simulink model "test_FOPID"  (R2024a)
settings: Solver=VariableStepAuto  StartTime=0.0  StopTime=0.1  RelTol=1e-3
undefined symbols (not defined in the file or in its folder): control_a, control_p, force_a, force_p, rpm_a, rpm_p
libraries: fod x145, slpidlib x15
(part 4 of 4)

== system test_FOPID/FOPID/ISE/Subsystem/TRAS 2_dof model 2/r(x2,x6) ==
  y2 : Inport
  x6 : Inport  Port=2
  +2 : Sum  InputSameDT=on  SaturateOnIntegerOverflow=on  OutDataTypeStr=Inherit: Same as first input
  Mux : Mux  Inputs=2
  r2 : Fcn  Expr=- ( 0.0292*cos(u)+ 0.0546*sin(u))*1.7143
  s : Fcn  Expr="(u(1)^2)*(     -0.07389953104162*  0.28753198180218*sin(u(2))*cos(u(2)))"
  r : Outport
  wires:
  Mux/1 -> s/1
  r2/1 -> +2/1
  s/1 -> +2/2
  x6/1 -> Mux/2, r2/1
  +2/1 -> r/1
  y2/1 -> Mux/1

== system test_FOPID/FOPID/ITAE/Subsystem/TRAS 2_dof model 2/DCP-azimuth ==
  CTR_A : Inport
  1/Ja : Gain  Gain=37000  SaturateOnIntegerOverflow=on  OutDataTypeStr=Inherit: Same as input  ParamDataTypeStr=Inherit: Same as input
  CtrlA(rpma) : Lookup  InputValues=rpm_a  Table=control_a
  Integrator1 : Integrator
  Sum1 : Sum  Inputs=|+-  InputSameDT=on  SaturateOnIntegerOverflow=on  OutDataTypeStr=Inherit: Same as first input
  forceA(rpma) : Lookup  InputValues=rpm_a  Table=force_a
  RPM_A : Outport
  FORCE_A : Outport  Port=2
  wires:
  Sum1/1 -> Integrator1/1
  CtrlA(rpma)/1 -> Sum1/2
  Integrator1/1 -> 1/Ja/1
  1/Ja/1 -> CtrlA(rpma)/1, forceA(rpma)/1, RPM_A/1
  CTR_A/1 -> Sum1/1
  forceA(rpma)/1 -> FORCE_A/1

== system test_FOPID/FOPID/ITAE/Subsystem/TRAS 2_dof model 2/DCP_pith ==
  CTR_P : Inport
  1/Jp1 : Gain  Gain=6100  OutDataTypeStr=Inherit: Same as input  ParamDataTypeStr=Inherit: Same as input
  CtrlP(rpmp) : Lookup  InputValues=rpm_p  Table=control_p
  Integrator : Integrator
  Sum : Sum  Inputs=|+-  InputSameDT=on  SaturateOnIntegerOverflow=on  OutDataTypeStr=Inherit: Same as first input
  force(rpmp) : Lookup  InputValues=rpm_p  Table=force_p
  RPM_P : Outport
  FORCE_P : Outport  Port=2
  wires:
  Sum/1 -> Integrator/1
  Integrator/1 -> 1/Jp1/1
  CtrlP(rpmp)/1 -> Sum/2
  1/Jp1/1 -> RPM_P/1, CtrlP(rpmp)/1, force(rpmp)/1
  CTR_P/1 -> Sum/1
  force(rpmp)/1 -> FORCE_P/1

== system test_FOPID/FOPID/ITAE/Subsystem/TRAS 2_dof model 2/q (x2,x6) ==
  x2 : Inport
  x6 : Inport  Port=2
  " q(x6)" : Fcn  Expr=( (0.0268-0.00300962066650)*cos(u)^2) +0.00300962066650
  *1 : Product  Inputs=*/  InputSameDT=on  SaturateOnIntegerOverflow=on  OutDataTypeStr=Inherit: Same as first input
  q : Outport
  wires:
  *1/1 -> q/1
  x2/1 -> *1/1
  x6/1 -> " q(x6)"/1
  " q(x6)"/1 -> *1/2

== system test_FOPID/FOPID/ITAE/Subsystem/TRAS 2_dof model 2/r(x2,x6) ==
  y2 : Inport
  x6 : Inport  Port=2
  +2 : Sum  InputSameDT=on  SaturateOnIntegerOverflow=on  OutDataTypeStr=Inherit: Same as first input
  Mux : Mux  Inputs=2
  r2 : Fcn  Expr=- ( 0.0292*cos(u)+ 0.0546*sin(u))*1.7143
  s : Fcn  Expr="(u(1)^2)*(     -0.07389953104162*  0.28753198180218*sin(u(2))*cos(u(2)))"
  r : Outport
  wires:
  Mux/1 -> s/1
  r2/1 -> +2/1
  s/1 -> +2/2
  x6/1 -> Mux/2, r2/1
  +2/1 -> r/1
  y2/1 -> Mux/1

== system test_FOPID/FOPID/ITSE/Subsystem/TRAS 2_dof model 2/DCP-azimuth ==
  CTR_A : Inport
  1/Ja : Gain  Gain=37000  SaturateOnIntegerOverflow=on  OutDataTypeStr=Inherit: Same as input  ParamDataTypeStr=Inherit: Same as input
  CtrlA(rpma) : Lookup  InputValues=rpm_a  Table=control_a
  Integrator1 : Integrator
  Sum1 : Sum  Inputs=|+-  InputSameDT=on  SaturateOnIntegerOverflow=on  OutDataTypeStr=Inherit: Same as first input
  forceA(rpma) : Lookup  InputValues=rpm_a  Table=force_a
  RPM_A : Outport
  FORCE_A : Outport  Port=2
  wires:
  Sum1/1 -> Integrator1/1
  CtrlA(rpma)/1 -> Sum1/2
  Integrator1/1 -> 1/Ja/1
  1/Ja/1 -> CtrlA(rpma)/1, forceA(rpma)/1, RPM_A/1
  CTR_A/1 -> Sum1/1
  forceA(rpma)/1 -> FORCE_A/1

== system test_FOPID/FOPID/ITSE/Subsystem/TRAS 2_dof model 2/DCP_pith ==
  CTR_P : Inport
  1/Jp1 : Gain  Gain=6100  OutDataTypeStr=Inherit: Same as input  ParamDataTypeStr=Inherit: Same as input
  CtrlP(rpmp) : Lookup  InputValues=rpm_p  Table=control_p
  Integrator : Integrator
  Sum : Sum  Inputs=|+-  InputSameDT=on  SaturateOnIntegerOverflow=on  OutDataTypeStr=Inherit: Same as first input
  force(rpmp) : Lookup  InputValues=rpm_p  Table=force_p
  RPM_P : Outport
  FORCE_P : Outport  Port=2
  wires:
  Sum/1 -> Integrator/1
  Integrator/1 -> 1/Jp1/1
  CtrlP(rpmp)/1 -> Sum/2
  1/Jp1/1 -> RPM_P/1, CtrlP(rpmp)/1, force(rpmp)/1
  CTR_P/1 -> Sum/1
  force(rpmp)/1 -> FORCE_P/1

== system test_FOPID/FOPID/ITSE/Subsystem/TRAS 2_dof model 2/q (x2,x6) ==
  x2 : Inport
  x6 : Inport  Port=2
  " q(x6)" : Fcn  Expr=( (0.0268-0.00300962066650)*cos(u)^2) +0.00300962066650
  *1 : Product  Inputs=*/  InputSameDT=on  SaturateOnIntegerOverflow=on  OutDataTypeStr=Inherit: Same as first input
  q : Outport
  wires:
  *1/1 -> q/1
  x2/1 -> *1/1
  x6/1 -> " q(x6)"/1
  " q(x6)"/1 -> *1/2

== system test_FOPID/FOPID/ITSE/Subsystem/TRAS 2_dof model 2/r(x2,x6) ==
  y2 : Inport
  x6 : Inport  Port=2
  +2 : Sum  InputSameDT=on  SaturateOnIntegerOverflow=on  OutDataTypeStr=Inherit: Same as first input
  Mux : Mux  Inputs=2
  r2 : Fcn  Expr=- ( 0.0292*cos(u)+ 0.0546*sin(u))*1.7143
  s : Fcn  Expr="(u(1)^2)*(     -0.07389953104162*  0.28753198180218*sin(u(2))*cos(u(2)))"
  r : Outport
  wires:
  Mux/1 -> s/1
  r2/1 -> +2/1
  s/1 -> +2/2
  x6/1 -> Mux/2, r2/1
  +2/1 -> r/1
  y2/1 -> Mux/1

== system test_FOPID/FOPID/sensibility/Subsystem/TRAS 2_dof model 3/DCP-azimuth ==
  CTR_A : Inport
  1/Ja : Gain  Gain=37000  SaturateOnIntegerOverflow=on  OutDataTypeStr=Inherit: Same as input  ParamDataTypeStr=Inherit: Same as input
  CtrlA(rpma) : Lookup  InputValues=rpm_a  Table=control_a
  Integrator1 : Integrator
  Sum1 : Sum  Inputs=|+-  InputSameDT=on  SaturateOnIntegerOverflow=on  OutDataTypeStr=Inherit: Same as first input
  forceA(rpma) : Lookup  InputValues=rpm_a  Table=force_a
  RPM_A : Outport
  FORCE_A : Outport  Port=2
  wires:
  forceA(rpma)/1 -> FORCE_A/1
  CTR_A/1 -> Sum1/1
  1/Ja/1 -> RPM_A/1, forceA(rpma)/1, CtrlA(rpma)/1
  Integrator1/1 -> 1/Ja/1
  CtrlA(rpma)/1 -> Sum1/2
  Sum1/1 -> Integrator1/1

== system test_FOPID/FOPID/sensibility/Subsystem/TRAS 2_dof model 3/DCP_pith ==
  CTR_P : Inport
  1/Jp1 : Gain  Gain=6100  OutDataTypeStr=Inherit: Same as input  ParamDataTypeStr=Inherit: Same as input
  CtrlP(rpmp) : Lookup  InputValues=rpm_p  Table=control_p
  Integrator : Integrator
  Sum : Sum  Inputs=|+-  InputSameDT=on  SaturateOnIntegerOverflow=on  OutDataTypeStr=Inherit: Same as first input
  force(rpmp) : Lookup  InputValues=rpm_p  Table=force_p
  RPM_P : Outport
  FORCE_P : Outport  Port=2
  wires:
  force(rpmp)/1 -> FORCE_P/1
  CTR_P/1 -> Sum/1
  1/Jp1/1 -> force(rpmp)/1, CtrlP(rpmp)/1, RPM_P/1
  CtrlP(rpmp)/1 -> Sum/2
  Integrator/1 -> 1/Jp1/1
  Sum/1 -> Integrator/1

== system test_FOPID/FOPID/sensibility/Subsystem/TRAS 2_dof model 3/q (x2,x6) ==
  x2 : Inport
  x6 : Inport  Port=2
  " q(x6)" : Fcn  Expr=( (0.0268-0.00300962066650)*cos(u)^2) +0.00300962066650
  *1 : Product  Inputs=*/  InputSameDT=on  SaturateOnIntegerOverflow=on  OutDataTypeStr=Inherit: Same as first input
  q : Outport
  wires:
  " q(x6)"/1 -> *1/2
  x6/1 -> " q(x6)"/1
  x2/1 -> *1/1
  *1/1 -> q/1

== system test_FOPID/FOPID/sensibility/Subsystem/TRAS 2_dof model 3/r(x2,x6) ==
  y2 : Inport
  x6 : Inport  Port=2
  +2 : Sum  InputSameDT=on  SaturateOnIntegerOverflow=on  OutDataTypeStr=Inherit: Same as first input
  Mux : Mux  Inputs=2
  r2 : Fcn  Expr=- ( 0.0292*cos(u)+ 0.0546*sin(u))*1.7143
  s : Fcn  Expr="(u(1)^2)*(     -0.07389953104162*  0.28753198180218*sin(u(2))*cos(u(2)))"
  r : Outport
  wires:
  y2/1 -> Mux/1
  +2/1 -> r/1
  x6/1 -> r2/1, Mux/2
  s/1 -> +2/2
  r2/1 -> +2/1
  Mux/1 -> s/1
